simulink model "MANUFACTURINGCELLInitial2"  (R2026a)
settings: Solver=VariableStepAuto  StopTime=20000.0
undefined symbols (not defined in the file): m, n
settings Model: Creator=Sayandip Mallick  LastModifiedBy=soumy

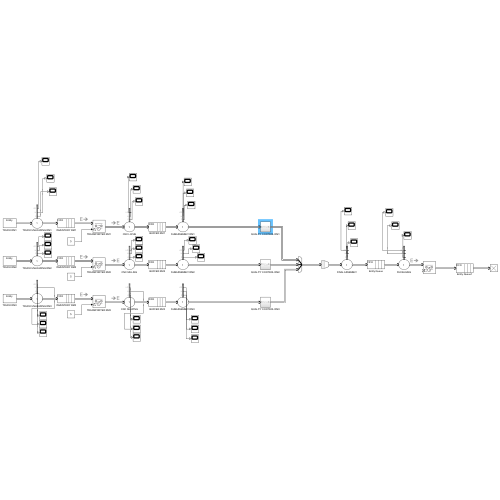
[thumbnail: Simulink's stored preview of the top-level diagram]
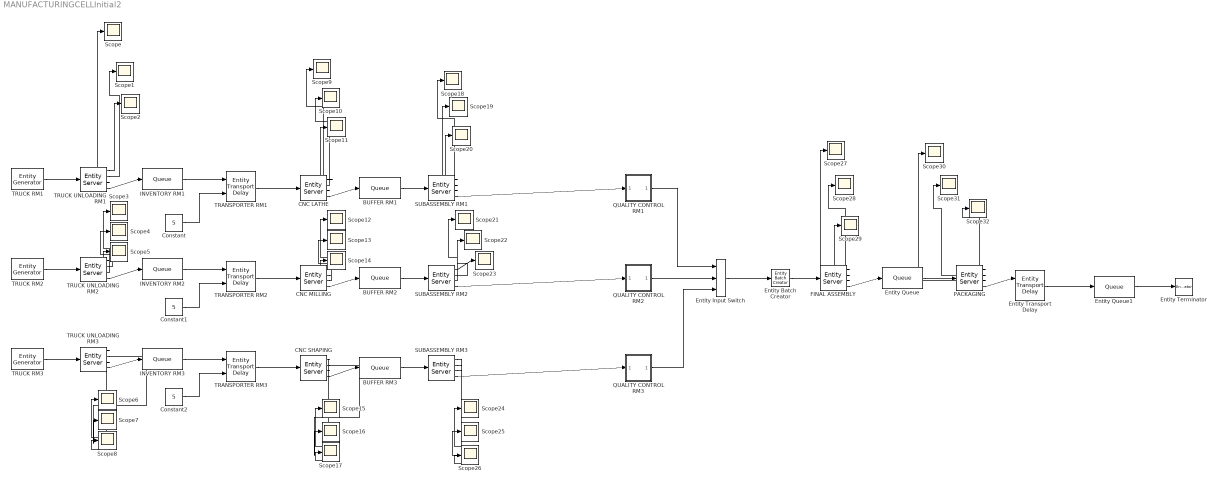
== system MANUFACTURINGCELLInitial2 ==
  BUFFER RM1 : Queue  InputPortMessageModes=m  OutputPortMessageModes=m
  BUFFER RM2 : Queue  InputPortMessageModes=m  OutputPortMessageModes=m
  BUFFER RM3 : Queue  InputPortMessageModes=m  OutputPortMessageModes=m
  CNC LATHE : EntityServer  InputPortMessageModes=m  OutputPortMessageModes=n,n,n,m  Capacity=1  ServiceTimeSource=MATLAB action  ServiceTimeAction=|  NumberEntitiesDeparted=on  AverageWait=on  Utilization=on
      | if rand(1,1) < 0.04
      |     dt = 60 + 30*rand(1,1);   % breakdown: 60-90 min downtime
      | else
      |     dt = -2*sum(log(rand(9,1)));        % normal machining time
      | end
      settings: OutputPortMap=o0,o4,o5,o9
  CNC MILLING : EntityServer  InputPortMessageModes=m  OutputPortMessageModes=n,n,n,m  Capacity=1  ServiceTimeSource=MATLAB action  ServiceTimeAction=|  NumberEntitiesDeparted=on  AverageWait=on  Utilization=on
      | if rand(1,1) < 0.04
      |     dt = 60 + 30*rand(1,1);   % breakdown: 60-90 min downtime
      | else
      |     dt = -2*sum(log(rand(9,1)));        % normal machining time
      | end
      settings: OutputPortMap=o0,o4,o5,o9
  CNC SHAPING : EntityServer  InputPortMessageModes=m  OutputPortMessageModes=n,n,n,m  Capacity=1  ServiceTimeSource=MATLAB action  ServiceTimeAction=|  NumberEntitiesDeparted=on  AverageWait=on  Utilization=on
      | if rand(1,1) < 0.04
      |     dt = 60 + 30*rand(1,1);   % breakdown: 60-90 min downtime
      | else
      |     dt = -2*sum(log(rand(9,1)));       % normal machining time
      | end
      settings: OutputPortMap=o0,o4,o5,o9
  Constant : Constant  Value=5
  Constant1 : Constant  Value=5
  Constant2 : Constant  Value=5
  Entity Input Switch : EntityInputSwitch  InputPortMessageModes=m,m,m  OutputPortMessageModes=m  NumberInputPorts=3
      settings: InputPortMap=u1,u2,u3
  Entity Transport Delay : EntityTransportDelay  InputPortMessageModes=m,n  OutputPortMessageModes=m
  Entity Batch Creator : EntityBatchCreator  InputPortMessageModes=m  OutputPortMessageModes=m  NumberOfEntitiesInBatch=3
      settings: OutputPortMap=o4
  Entity Queue : Queue  InputPortMessageModes=m  OutputPortMessageModes=m
  Entity Queue1 : Queue  InputPortMessageModes=m  OutputPortMessageModes=m
  Entity Terminator : EntityTerminator  InputPortMessageModes=m
  FINAL ASSEMBLY : EntityServer  InputPortMessageModes=m  OutputPortMessageModes=n,n,n,m  Capacity=1  ServiceTimeSource=MATLAB action  ServiceTimeAction=dt = max(20 + 4*randn(1,1), 1);  NumberEntitiesDeparted=on  AverageWait=on  Utilization=on
      settings: OutputPortMap=o0,o4,o5,o9
  INVENTORY RM1 : Queue  InputPortMessageModes=m  OutputPortMessageModes=m
  INVENTORY RM2 : Queue  InputPortMessageModes=m  OutputPortMessageModes=m
  INVENTORY RM3 : Queue  InputPortMessageModes=m  OutputPortMessageModes=m
  PACKAGING : EntityServer  InputPortMessageModes=m  OutputPortMessageModes=n,n,n,m  Capacity=1  ServiceTimeSource=MATLAB action  ServiceTimeAction=dt = 5 + 1*rand(1,1);  NumberEntitiesDeparted=on  AverageWait=on  Utilization=on
      settings: OutputPortMap=o0,o4,o5,o9
  QUALITY CONTROL RM1 : Subsystem
  QUALITY CONTROL RM2 : Subsystem
  QUALITY CONTROL RM3 : Subsystem
  SUBASSEMBLY RM1 : EntityServer  InputPortMessageModes=m  OutputPortMessageModes=n,n,n,m  Capacity=1  ServiceTimeSource=MATLAB action  ServiceTimeAction=dt = max(12 + 3*randn(1,1), 1);  NumberEntitiesDeparted=on  AverageWait=on  Utilization=on
      settings: OutputPortMap=o0,o4,o5,o9
  SUBASSEMBLY RM2 : EntityServer  InputPortMessageModes=m  OutputPortMessageModes=n,n,n,m  Capacity=1  ServiceTimeSource=MATLAB action  ServiceTimeAction=dt = max(12 + 3*randn(1,1), 1);  NumberEntitiesDeparted=on  AverageWait=on  Utilization=on
      settings: OutputPortMap=o0,o4,o5,o9
  SUBASSEMBLY RM3 : EntityServer  InputPortMessageModes=m  OutputPortMessageModes=n,n,n,m  Capacity=1  ServiceTimeSource=MATLAB action  ServiceTimeAction=dt = max(12 + 3*randn(1,1), 1);  NumberEntitiesDeparted=on  AverageWait=on  Utilization=on
      settings: OutputPortMap=o0,o4,o5,o9
  Scope{,1..32} (33 alike) : Scope
      Scope settings: ActiveDisplayYMinimum=-0.033961298022833139  ActiveDisplayYMaximum=0.67498053084519971
      Scope1 settings: ActiveDisplayYMinimum=8.9964886004213565  ActiveDisplayYMaximum=9.8009630704740545
      Scope10 settings: ActiveDisplayYMinimum=9.88821648505752  ActiveDisplayYMaximum=22.982550291701781  DataLoggingVariableName=ScopeData10
      Scope11 settings: ActiveDisplayYMinimum=-7.2499999999999982  ActiveDisplayYMaximum=75.25  DataLoggingVariableName=ScopeData11
      Scope12 settings: ActiveDisplayYMinimum=-0.052037915664992523  ActiveDisplayYMaximum=0.46834124098493285  DataLoggingVariableName=ScopeData12
      Scope13 settings: ActiveDisplayYMinimum=9.88821648505752  ActiveDisplayYMaximum=22.982550291701781  DataLoggingVariableName=ScopeData13
      Scope14 settings: ActiveDisplayYMinimum=-7.2499999999999982  ActiveDisplayYMaximum=75.25  DataLoggingVariableName=ScopeData14
      Scope15 settings: ActiveDisplayYMinimum=-0.052037915664992523  ActiveDisplayYMaximum=0.46834124098493285  DataLoggingVariableName=ScopeData15
      Scope16 settings: ActiveDisplayYMinimum=9.88821648505752  ActiveDisplayYMaximum=22.982550291701781  DataLoggingVariableName=ScopeData16
      Scope17 settings: ActiveDisplayYMinimum=-7.2499999999999982  ActiveDisplayYMaximum=75.25  DataLoggingVariableName=ScopeData17
      Scope18 settings: ActiveDisplayYMinimum=-0.040282268719271791  ActiveDisplayYMaximum=0.3625404184734462  DataLoggingVariableName=ScopeData18
      Scope19 settings: ActiveDisplayYMinimum=11.339509246783336  ActiveDisplayYMaximum=16.025974785037164  DataLoggingVariableName=ScopeData19
      Scope2 settings: ActiveDisplayYMinimum=-7.2499999999999982  ActiveDisplayYMaximum=75.25  DataLoggingVariableName=ScopeData2
      Scope20 settings: ActiveDisplayYMinimum=-7.2499999999999982  ActiveDisplayYMaximum=75.25  DataLoggingVariableName=ScopeData20
      Scope21 settings: ActiveDisplayYMinimum=-0.036018921286554387  ActiveDisplayYMaximum=0.32417029157898952  DataLoggingVariableName=ScopeData21
      Scope22 settings: DataLoggingVariableName=ScopeData22
      Scope23 settings: DataLoggingVariableName=ScopeData23
      Scope24 settings: DataLoggingVariableName=ScopeData24
      Scope25 settings: DataLoggingVariableName=ScopeData25
      Scope26 settings: DataLoggingVariableName=ScopeData26
      Scope27 settings: ActiveDisplayYMinimum=-0.0093313046534982038  ActiveDisplayYMaximum=0.083981741881483857  DataLoggingVariableName=ScopeData27
      Scope28 settings: ActiveDisplayYMinimum=19.119345662377782  ActiveDisplayYMaximum=25.367966380049577  DataLoggingVariableName=ScopeData28
      Scope29 settings: ActiveDisplayYMinimum=-6.7499999999999982  ActiveDisplayYMaximum=70.75  DataLoggingVariableName=ScopeData29
      Scope3 settings: ActiveDisplayYMinimum=-0.090961489822150132  ActiveDisplayYMaximum=1.1212179433135723  DataLoggingVariableName=ScopeData3
      Scope30 settings: ActiveDisplayYMinimum=-0.0023309211253362844  ActiveDisplayYMaximum=0.020978290128026565  DataLoggingVariableName=ScopeData30
      Scope31 settings: ActiveDisplayYMinimum=5.49824430021064  ActiveDisplayYMaximum=5.9004815352370237  DataLoggingVariableName=ScopeData31
      Scope32 settings: ActiveDisplayYMinimum=-6.7499999999999982  ActiveDisplayYMaximum=70.75  DataLoggingVariableName=ScopeData32
      Scope4 settings: ActiveDisplayYMinimum=8.9964886004213565  ActiveDisplayYMaximum=9.8009630704740545  DataLoggingVariableName=ScopeData4
      Scope5 settings: ActiveDisplayYMinimum=-7.2499999999999982  ActiveDisplayYMaximum=75.25  DataLoggingVariableName=ScopeData5
      Scope6 settings: DataLoggingVariableName=ScopeData6
      Scope7 settings: DataLoggingVariableName=ScopeData7
      Scope8 settings: DataLoggingVariableName=ScopeData8
      Scope9 settings: ActiveDisplayYMinimum=-0.061126068308985017  ActiveDisplayYMaximum=0.55013461478086523  DataLoggingVariableName=ScopeData9
  TRANSPORTER RM1 : EntityTransportDelay  InputPortMessageModes=m,n  OutputPortMessageModes=m
  TRANSPORTER RM2 : EntityTransportDelay  InputPortMessageModes=m,n  OutputPortMessageModes=m
  TRANSPORTER RM3 : EntityTransportDelay  InputPortMessageModes=m,n  OutputPortMessageModes=m
  TRUCK RM1 : EntityGenerator  OutputPortMessageModes=m  Period=300  AttributeName=Attribute1|Attribute2|Attribute3  AttributeInitialValue=0|0|0  EntityType=Structured  EntityTypeName=Entity
  TRUCK RM2 : EntityGenerator  OutputPortMessageModes=m  Period=300  AttributeName=Attribute1|Attribute2|Attribute3  AttributeInitialValue=0|0|0  EntityType=Structured  EntityTypeName=Entity
  TRUCK RM3 : EntityGenerator  OutputPortMessageModes=m  Period=300  AttributeName=Attribute1|Attribute2|Attribute3  AttributeInitialValue=0|0|0  EntityType=Structured  EntityTypeName=Entity
  TRUCK UNLOADING RM1 : EntityServer  InputPortMessageModes=m  OutputPortMessageModes=n,n,n,m  Capacity=1  ServiceTimeSource=MATLAB action  ServiceTimeAction=dt = 8 + 2*rand(1,1);  NumberEntitiesDeparted=on  AverageWait=on  Utilization=on
      settings: OutputPortMap=o0,o4,o5,o9
  TRUCK UNLOADING RM2 : EntityServer  InputPortMessageModes=m  OutputPortMessageModes=n,n,n,m  Capacity=1  ServiceTimeSource=MATLAB action  ServiceTimeAction=dt = 8 + 2*rand(1,1);  NumberEntitiesDeparted=on  AverageWait=on  Utilization=on
      settings: OutputPortMap=o0,o4,o5,o9
  TRUCK UNLOADING RM3 : EntityServer  InputPortMessageModes=m  OutputPortMessageModes=n,n,n,m  Capacity=1  ServiceTimeSource=MATLAB action  ServiceTimeAction=dt = 8 + 2*rand(1,1);  NumberEntitiesDeparted=on  AverageWait=on  Utilization=on
      settings: OutputPortMap=o0,o4,o5,o9
  wires:
  TRUCK RM1/1 -> TRUCK UNLOADING RM1/1
  TRUCK UNLOADING RM1/4 -> INVENTORY RM1/1
  INVENTORY RM1/1 -> TRANSPORTER RM1/1
  TRANSPORTER RM1/1 -> CNC LATHE/1
  TRANSPORTER RM2/1 -> CNC MILLING/1
  TRUCK UNLOADING RM2/4 -> INVENTORY RM2/1
  TRUCK RM2/1 -> TRUCK UNLOADING RM2/1
  INVENTORY RM2/1 -> TRANSPORTER RM2/1
  TRANSPORTER RM3/1 -> CNC SHAPING/1
  TRUCK UNLOADING RM3/4 -> INVENTORY RM3/1
  TRUCK RM3/1 -> TRUCK UNLOADING RM3/1
  INVENTORY RM3/1 -> TRANSPORTER RM3/1
  Constant/1 -> TRANSPORTER RM1/2
  Constant1/1 -> TRANSPORTER RM2/2
  Constant2/1 -> TRANSPORTER RM3/2
  CNC LATHE/4 -> BUFFER RM1/1
  CNC MILLING/4 -> BUFFER RM2/1
  CNC SHAPING/4 -> BUFFER RM3/1
  BUFFER RM1/1 -> SUBASSEMBLY RM1/1
  BUFFER RM2/1 -> SUBASSEMBLY RM2/1
  BUFFER RM3/1 -> SUBASSEMBLY RM3/1
  SUBASSEMBLY RM1/4 -> QUALITY CONTROL RM1/1(In1)
  SUBASSEMBLY RM2/4 -> QUALITY CONTROL RM2/1(In1)
  SUBASSEMBLY RM3/4 -> QUALITY CONTROL RM3/1(In1)
  QUALITY CONTROL RM1/1(Out1) -> Entity Input Switch/1
  QUALITY CONTROL RM2/1(Out1) -> Entity Input Switch/2
  QUALITY CONTROL RM3/1(Out1) -> Entity Input Switch/3
  Entity Input Switch/1 -> Entity Batch Creator/1
  Entity Batch Creator/1 -> FINAL ASSEMBLY/1
  FINAL ASSEMBLY/4 -> Entity Queue/1
  Entity Queue/1 -> PACKAGING/1
  PACKAGING/4 -> Entity Transport Delay/1
  Entity Transport Delay/1 -> Entity Queue1/1
  Entity Queue1/1 -> Entity Terminator/1
  TRUCK UNLOADING RM1/3 -> Scope/1
  TRUCK UNLOADING RM1/2 -> Scope1/1
  TRUCK UNLOADING RM1/1 -> Scope2/1
  TRUCK UNLOADING RM2/3 -> Scope3/1
  TRUCK UNLOADING RM2/2 -> Scope4/1
  TRUCK UNLOADING RM2/1 -> Scope5/1
  TRUCK UNLOADING RM3/3 -> Scope6/1
  TRUCK UNLOADING RM3/2 -> Scope7/1
  TRUCK UNLOADING RM3/1 -> Scope8/1
  CNC MILLING/3 -> Scope12/1
  CNC MILLING/2 -> Scope13/1
  CNC MILLING/1 -> Scope14/1
  CNC LATHE/3 -> Scope9/1
  CNC LATHE/2 -> Scope10/1
  CNC LATHE/1 -> Scope11/1
  CNC SHAPING/3 -> Scope15/1
  CNC SHAPING/2 -> Scope16/1
  CNC SHAPING/1 -> Scope17/1
  SUBASSEMBLY RM1/3 -> Scope18/1
  SUBASSEMBLY RM1/2 -> Scope19/1
  SUBASSEMBLY RM1/1 -> Scope20/1
  SUBASSEMBLY RM2/3 -> Scope21/1
  SUBASSEMBLY RM2/2 -> Scope22/1
  SUBASSEMBLY RM2/1 -> Scope23/1
  SUBASSEMBLY RM3/3 -> Scope24/1
  SUBASSEMBLY RM3/2 -> Scope25/1
  SUBASSEMBLY RM3/1 -> Scope26/1
  FINAL ASSEMBLY/3 -> Scope27/1
  FINAL ASSEMBLY/2 -> Scope28/1
  FINAL ASSEMBLY/1 -> Scope29/1
  PACKAGING/3 -> Scope30/1
  PACKAGING/2 -> Scope31/1
  PACKAGING/1 -> Scope32/1

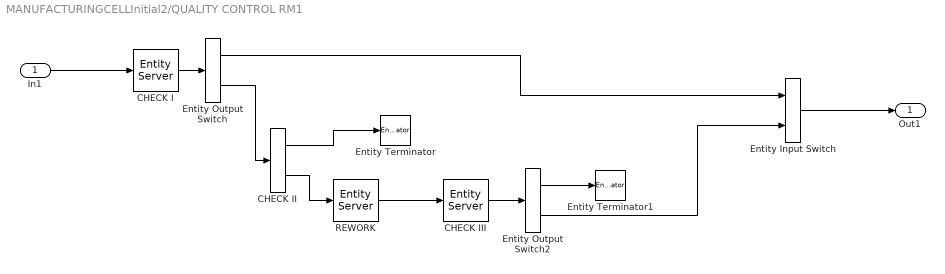
== system MANUFACTURINGCELLInitial2/QUALITY CONTROL RM1 ==
  In1 : Inport
  CHECK I : EntityServer  InputPortMessageModes=m  OutputPortMessageModes=m  Capacity=1  ServiceTimeSource=MATLAB action  ServiceTimeAction=dt = 3 + 1*rand(1,1);  ServiceCompleteAction=|
      | r1 = rand(1,1);
      | if r1 < 0.90
      |     entity.Attribute1 = 1;   % 90%% pass first inspection
      | else
      |     entity.Attribute1 = 2;   % 10%% flagged for second check
      | end
      | r2 = rand(1,1);
      | if r2 < 0.25
      |     entity.Attribute2 = 1;   % of flagged items, 25%% unfixable -> scrap
      | else
      |     entity.Attribute2 = 2;   % 75%% sent to rework
      | end
  CHECK II : EntityOutputSwitch  InputPortMessageModes=m  OutputPortMessageModes=m,m  SwitchingCriterion=From attribute  SwitchAttributeName=Attribute2
  CHECK III : EntityServer  InputPortMessageModes=m  OutputPortMessageModes=m  Capacity=1  ServiceTimeSource=MATLAB action  ServiceTimeAction=dt = 2 + 0.5*rand(1,1);  ServiceCompleteAction=|
      | r3 = rand(1,1);
      | if r3 < 0.15
      |     entity.Attribute3 = 1;   % rework failed -> scrap
      | else
      |     entity.Attribute3 = 2;   % rework succeeded -> merge to output
      | end
  Entity Input Switch : EntityInputSwitch  InputPortMessageModes=m,m  OutputPortMessageModes=m
  Entity Output Switch : EntityOutputSwitch  InputPortMessageModes=m  OutputPortMessageModes=m,m  SwitchingCriterion=From attribute  SwitchAttributeName=Attribute1
  Entity Output Switch2 : EntityOutputSwitch  InputPortMessageModes=m  OutputPortMessageModes=m,m  SwitchingCriterion=From attribute  SwitchAttributeName=Attribute3
  Entity Terminator : EntityTerminator  InputPortMessageModes=m
  Entity Terminator1 : EntityTerminator  InputPortMessageModes=m
  REWORK : EntityServer  InputPortMessageModes=m  OutputPortMessageModes=m  Capacity=1  ServiceTimeSource=MATLAB action  ServiceTimeAction=dt = 15 + 5*rand(1,1);
  Out1 : Outport
  wires:
  Entity Output Switch/2 -> CHECK II/1
  CHECK II/2 -> REWORK/1
  CHECK III/1 -> Entity Output Switch2/1
  Entity Output Switch2/1 -> Entity Terminator1/1
  CHECK I/1 -> Entity Output Switch/1
  REWORK/1 -> CHECK III/1
  CHECK II/1 -> Entity Terminator/1
  In1/1 -> CHECK I/1
  Entity Output Switch/1 -> Entity Input Switch/1
  Entity Output Switch2/2 -> Entity Input Switch/2
  Entity Input Switch/1 -> Out1/1

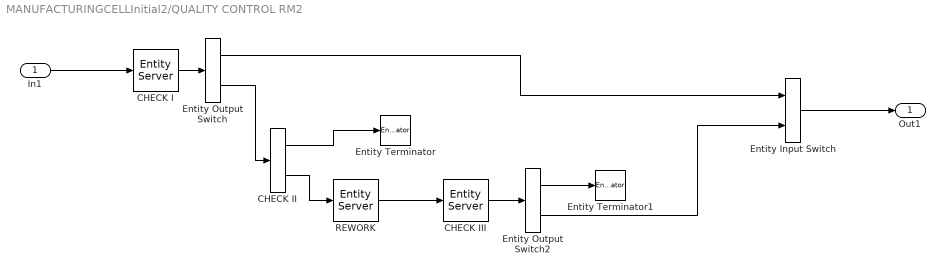
== system MANUFACTURINGCELLInitial2/QUALITY CONTROL RM2 ==
  In1 : Inport
  CHECK I : EntityServer  InputPortMessageModes=m  OutputPortMessageModes=m  Capacity=1  ServiceTimeSource=MATLAB action  ServiceTimeAction=dt = 3 + 1*rand(1,1);  ServiceCompleteAction=|
      | r1 = rand(1,1);
      | if r1 < 0.90
      |     entity.Attribute1 = 1;   % 90%% pass first inspection
      | else
      |     entity.Attribute1 = 2;   % 10%% flagged for second check
      | end
      | r2 = rand(1,1);
      | if r2 < 0.25
      |     entity.Attribute2 = 1;   % of flagged items, 25%% unfixable -> scrap
      | else
      |     entity.Attribute2 = 2;   % 75%% sent to rework
      | end
  CHECK II : EntityOutputSwitch  InputPortMessageModes=m  OutputPortMessageModes=m,m  SwitchingCriterion=From attribute  SwitchAttributeName=Attribute2
  CHECK III : EntityServer  InputPortMessageModes=m  OutputPortMessageModes=m  Capacity=1  ServiceTimeSource=MATLAB action  ServiceTimeAction=dt = 2 + 0.5*rand(1,1);  ServiceCompleteAction=|
      | r3 = rand(1,1);
      | if r3 < 0.15
      |     entity.Attribute3 = 1;   % rework failed -> scrap
      | else
      |     entity.Attribute3 = 2;   % rework succeeded -> merge to output
      | end
  Entity Input Switch : EntityInputSwitch  InputPortMessageModes=m,m  OutputPortMessageModes=m
  Entity Output Switch : EntityOutputSwitch  InputPortMessageModes=m  OutputPortMessageModes=m,m  SwitchingCriterion=From attribute  SwitchAttributeName=Attribute1
  Entity Output Switch2 : EntityOutputSwitch  InputPortMessageModes=m  OutputPortMessageModes=m,m  SwitchingCriterion=From attribute  SwitchAttributeName=Attribute3
  Entity Terminator : EntityTerminator  InputPortMessageModes=m
  Entity Terminator1 : EntityTerminator  InputPortMessageModes=m
  REWORK : EntityServer  InputPortMessageModes=m  OutputPortMessageModes=m  Capacity=1  ServiceTimeSource=MATLAB action  ServiceTimeAction=dt = 15 + 5*rand(1,1);
  Out1 : Outport
  wires:
  Entity Output Switch/2 -> CHECK II/1
  CHECK II/2 -> REWORK/1
  CHECK III/1 -> Entity Output Switch2/1
  Entity Output Switch2/1 -> Entity Terminator1/1
  CHECK I/1 -> Entity Output Switch/1
  REWORK/1 -> CHECK III/1
  CHECK II/1 -> Entity Terminator/1
  In1/1 -> CHECK I/1
  Entity Output Switch/1 -> Entity Input Switch/1
  Entity Output Switch2/2 -> Entity Input Switch/2
  Entity Input Switch/1 -> Out1/1

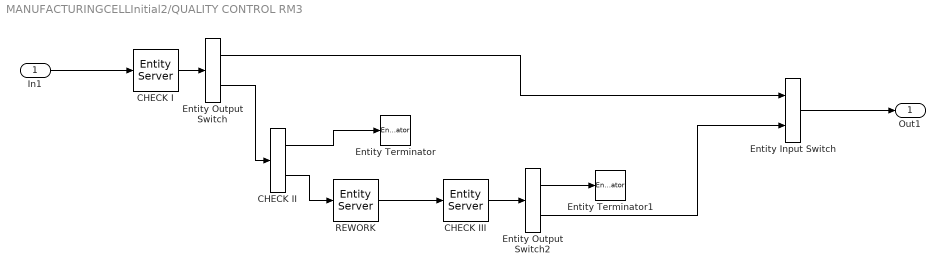
== system MANUFACTURINGCELLInitial2/QUALITY CONTROL RM3 ==
  In1 : Inport
  CHECK I : EntityServer  InputPortMessageModes=m  OutputPortMessageModes=m  Capacity=1  ServiceTimeSource=MATLAB action  ServiceTimeAction=dt = 3 + 1*rand(1,1);  ServiceCompleteAction=|
      | r1 = rand(1,1);
      | if r1 < 0.90
      |     entity.Attribute1 = 1;   % 90%% pass first inspection
      | else
      |     entity.Attribute1 = 2;   % 10%% flagged for second check
      | end
      | r2 = rand(1,1);
      | if r2 < 0.25
      |     entity.Attribute2 = 1;   % of flagged items, 25%% unfixable -> scrap
      | else
      |     entity.Attribute2 = 2;   % 75%% sent to rework
      | end
  CHECK II : EntityOutputSwitch  InputPortMessageModes=m  OutputPortMessageModes=m,m  SwitchingCriterion=From attribute  SwitchAttributeName=Attribute2
  CHECK III : EntityServer  InputPortMessageModes=m  OutputPortMessageModes=m  Capacity=1  ServiceTimeSource=MATLAB action  ServiceTimeAction=dt = 2 + 0.5*rand(1,1);  ServiceCompleteAction=|
      | r3 = rand(1,1);
      | if r3 < 0.15
      |     entity.Attribute3 = 1;   % rework failed -> scrap
      | else
      |     entity.Attribute3 = 2;   % rework succeeded -> merge to output
      | end
  Entity Input Switch : EntityInputSwitch  InputPortMessageModes=m,m  OutputPortMessageModes=m
  Entity Output Switch : EntityOutputSwitch  InputPortMessageModes=m  OutputPortMessageModes=m,m  SwitchingCriterion=From attribute  SwitchAttributeName=Attribute1
  Entity Output Switch2 : EntityOutputSwitch  InputPortMessageModes=m  OutputPortMessageModes=m,m  SwitchingCriterion=From attribute  SwitchAttributeName=Attribute3
  Entity Terminator : EntityTerminator  InputPortMessageModes=m
  Entity Terminator1 : EntityTerminator  InputPortMessageModes=m
  REWORK : EntityServer  InputPortMessageModes=m  OutputPortMessageModes=m  Capacity=1  ServiceTimeSource=MATLAB action  ServiceTimeAction=dt = 15 + 5*rand(1,1);
  Out1 : Outport
  wires:
  Entity Output Switch/2 -> CHECK II/1
  CHECK II/2 -> REWORK/1
  CHECK III/1 -> Entity Output Switch2/1
  Entity Output Switch2/1 -> Entity Terminator1/1
  CHECK I/1 -> Entity Output Switch/1
  REWORK/1 -> CHECK III/1
  CHECK II/1 -> Entity Terminator/1
  In1/1 -> CHECK I/1
  Entity Output Switch/1 -> Entity Input Switch/1
  Entity Output Switch2/2 -> Entity Input Switch/2
  Entity Input Switch/1 -> Out1/1
